simulink model "Controller_v2"  (R2015b)
settings: Solver=VariableStepAuto  StartTime=0.0  StopTime=10.0  RelTol=1e-3
settings Model: Creator=MVdB  LastModifiedBy=Niels

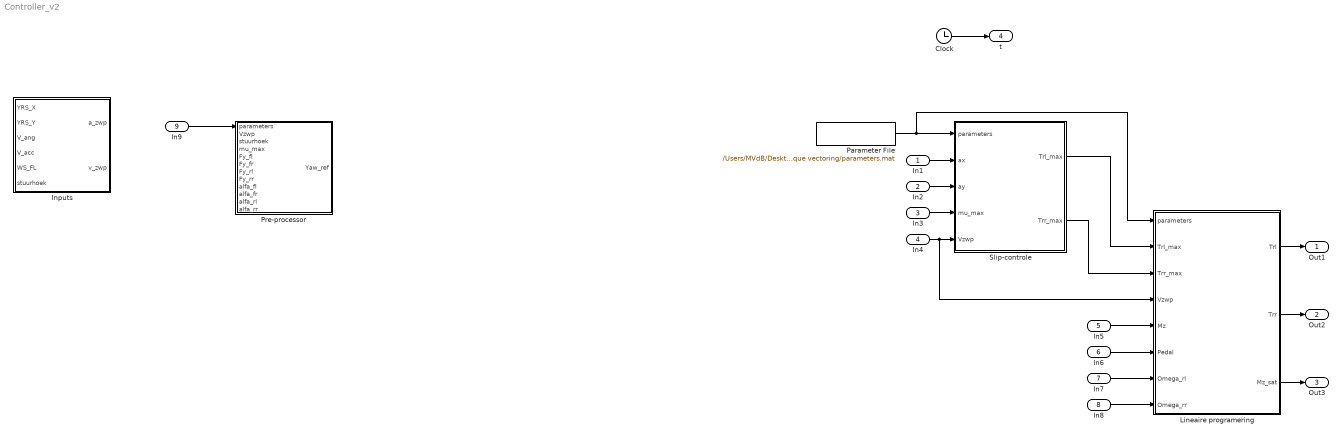
== system Controller_v2 ==
  In1 : Inport
  In2 : Inport  Port=2
  In3 : Inport  Port=3
  In4 : Inport  Port=4
  In5 : Inport  Port=5
  In6 : Inport  Port=6
  In7 : Inport  Port=7
  In8 : Inport  Port=8
  In9 : Inport  Port=9
  Clock : Clock
  Inputs : MATLAB Function  TreatAsAtomicUnit=on
  Lineaire programering : MATLAB Function  TreatAsAtomicUnit=on
  Parameter File : FromFile  FileName=/Users/MVdB/Desktop/FEB/Torque vectoring/parameters.mat  SampleTime=0
  Pre-processor : MATLAB Function  TreatAsAtomicUnit=on
  "Slip-controle " : MATLAB Function  TreatAsAtomicUnit=on
  Out1 : Outport
  Out2 : Outport  Port=2
  Out3 : Outport  Port=3
  t : Outport  Port=4
  wires:
  "Slip-controle "/2(Trr_max) -> Lineaire programering/3(Trr_max)
  "Slip-controle "/1(Trl_max) -> Lineaire programering/2(Trl_max)
  In1/1 -> "Slip-controle "/2(ax)
  In2/1 -> "Slip-controle "/3(ay)
  Lineaire programering/3(Mz_sat) -> Out3/1
  Lineaire programering/1(Trl) -> Out1/1
  Lineaire programering/2(Trr) -> Out2/1
  In3/1 -> "Slip-controle "/4(mu_max)
  In4/1 -> Lineaire programering/4(Vzwp), "Slip-controle "/5(Vzwp)
  In5/1 -> Lineaire programering/5(Mz)
  In6/1 -> Lineaire programering/6(Pedal)
  In7/1 -> Lineaire programering/7(Omega_rl)
  In8/1 -> Lineaire programering/8(Omega_rr)
  Clock/1 -> t/1
  Parameter File/1 -> Lineaire programering/1(parameters), "Slip-controle "/1(parameters)
  In9/1 -> Pre-processor/1(parameters)

== matlab function Controller_v2/Lineaire programering ==
  data: parameters input; Trl_max input; Trl output; Trr_max input; Vzwp input; Mz input; Pedal input; Omega_rl input; Omega_rr input; Trr output; Mz_sat output
function [Trl,Trr,Mz_sat] = Lineaire_programmering(parameters,Trl_max,Trr_max,Vzwp,Mz,Pedal,Omega_rl,Omega_rr)
%Deze blok staat in voor het berekenen van de te leveren torque per wiel
%aan de hand van twee lineaire doelen. Het eerste doel is het netto moment
%rond het zwaartepunt optimaliseren. Het tweede doel is de torque die wordt
%overgedragen op het wegdek optimaliseren.

%Gevraagd Moment
TV_control = (Mz*Reff_r)/(2*Sr*Gr);

TV_max_1 = min(400,((Trl_max+Trr_max)/2));


f = [Trr_1 Trl_1 e];
A = [Trr_1 Trl_1
    0];
b = [Tmax e];
Aeq = [Trr_1 -Trl_1 e];
beq = 2*max(-TV_max_1,min(TV_max_1,TV_control));
lb = [-Trr_1,-Trl_1];
ub = [Trr_1,Trl_1];

x = linprog(f,A,b,Aeq,beq,lb,ub);


%Gevraagde torque
TV_max_2 = max(0,min(400,(Trl_max-(Ttot/2)),(Trr_max+(Ttot/2))));

f_2 = [Trr_2 Trl_2];
A_2 = [Trr_2 Trl_2];
b_2 = Tmax;
Aeq_2 = [Trr_2 -Trl_2];
beq_2 = 2*max(-TV_max_2,min(TV_max_2,TV_control));
lb_2 = [-Trr_2,-Trl_2];
ub_2 = [Trr_2,Trl_2];

x_2  = linprog(f_2,A_2,b_2,Aeq_2,beq_2,lb_2,ub_2);


%Effectieve torques naar motordrives
Trl = x(2)*Cte + x_2(2)*(1-Cte);
Trr = x(1)*Cte + x_2(1)*(1-Cte);

== matlab function Controller_v2/Slip-controle  ==
  data: parameters input; ax input; ay input; mu_max input; Trl_max output; Vzwp input; Trr_max output
function [Trl_max,Trr_max] = Slip_controle(parameters,ax,ay,mu_max,Vzwp)
% Berekening van de maximale torques die men kan toepassen op de wielen
% door berekening van de normaalkrachten op de wielen.

load('parameters.mat');

%Wielbelastingen

%Statische wielbelasting
Ws_fl = (Lf/(2*L))*M*g;
Ws_fr = Ws_fl;
Ws_rl = (Lr/(2*L))*M*g;
Ws_rr = Ws_rl;

Ws_f = Ws_fl + Ws_fr;
Ws_r = Ws_rl + Ws_rr;

%Laterale wielbelasting (door rollen van de wagen)
FfsM = (Ksf*W*ay*D)/(Tf(Ksf+Ksr-(W*g*D)));   %Kracht door rolmoment
FrsM = (Ksr*W*ay*D)/(Tr(Ksf+Ksr-(W*g*D)));

FfsF = (Ws_f*ay*Hrcf)/Tf;                    %Kracht door afgeveerde massa
FrsF = (Ws_r*ay*Hrcr)/Tr;

FfuF = (Wu_f*ay*Hurcf)/Tf;                   %Kracht door onafgeveerde massa
FruF = (Wu_r*ay*Hurcr)/Tr;

Ff = FfsM + FfsF + FfuF;                    %Totale gewichtsverplaatsing
Fr = FrsM + FrsF + FruF;

Wy_fl = Ff/2;                               %Kracht per wiel
Wy_fr = -Wy_fl;
Wy_rl = Fr/2;
Wy_rr = -Wy_rl;

%Longitudinale wielbelasting
Wx_fl = (-H/(2*L))*W*ax;
Wx_fr = Wx_fl;
Wx_rl = (H/(2*L))*W*ax;
Wx_rr = Wx_rl;

%Aerodynamische wielbelasting
Wa_fl = (-LF/(2*L))+((Krf/(Krf+Krr))*(Rm/Tf));
Wa_fr = (-LF/(2*L))-((Krf/(Krf+Krr))*(Rm/Tf));
Wa_rl = (-LR/(2*L))+((Krr/(Krf+Krr))*(Rm/Tr));
Wa_rr = (-LR/(2*L))-((Krr/(Krf+Krr))*(Rm/Tr));

%anti-roll bar wielbelasting
Wab_fl = (Krf_a/((Krf_a+((Kwf*(Tf)^2)/2))*Wy_fl));
Wab_fr = -Wab_fl;
Wab_rl = (Krr_a/((Krr_a+((Kwr*(Tr)^2)/2))*Wy_rl));
Wab_rr = -Wab_rl;

%Totale belasting per wiel
Wfl = Ws_fl + Wy_fl + Wx_fl + Wa_fl + Wab_fl;   %Ongebruikt, kan later gebruikt worden voor 4WD
Wfr = Ws_fr + Wy_fr + Wx_fr + Wa_fr + Wab_fr;   %^ Idem
Wrl = Ws_rl + Wy_rl + Wx_rl + Wa_rl + Wab_rl;
Wrr = Ws_rr + Wy_rr + Wx_rr + Wa_rr + Wab_rr;



%Omrekening naar torques

%Wrijvingscirkels
Fx_rl = sqrt((Wrl^2*mu_max^2)-(Wrl^2*ay^2));
Fx_rr = sqrt((Wrr^2*mu_max^2)-(Wrr^2*ay^2));

%Maximum torques
Trl_max = Fx_rl*Reff_r;
Trr_max = Fx_rr*Reff_r;

== matlab function Controller_v2/Pre-processor ==
  data: parameters input; Yaw_ref output; Vzwp input; stuurhoek input; mu_max input; Fy_fl input; Fy_fr input; Fy_rl input; Fy_rr input; alfa_fl input; alfa_fr input; alfa_rl input; alfa_rr input
function Yaw_ref = pre_processor(parameters,Vzwp,stuurhoek,mu_max,Fy_fl,Fy_fr,Fy_rl,Fy_rr,alfa_fl,alfa_fr,alfa_rl,alfa_rr)
%De pre-processor berekend de gewenste yaw rate door het minimum te nemen
%van de ideale en de maximale yaw rate waarde.

%Berekening massa's
Mf = M*(Lr/L);
Mr = M*(Lf/L);

%Berekening Cornering stiffness
C_fl = (Fy_fl/alfa_fl);
C_fr = (Fy_fr/alfa_fr);
C_rl = (Fy_rl/alfa_rl);
C_rr = (Fy_rr/alfa_rr);

%Gemiddelde van de cornering stiffness vooraan en achteraan nemen
 Cf = ((C_fl + C_fr)/ 2);
 Cr = ((C_rl + C_rr)/ 2);
%Berekening van de onderstuur factor.
Ku = ((Mf/Cf)-(Mr/Cr));

%Berekening van de ideale yaw rate.
Yaw_id = ((Vzwp*stuurhoek)/((Lf+Lr)+Ku*(Vzwp)^2));

% berekening van de sliphoek beita
beita = atan(Lf * tan(stuurhoek)/ (Lf+Lr)) ;

%Berekening van de maximale yaw rate.
Yaw_max = ((mu_max*g)/(Vzwp*cos(beita)))-Vzwp*diff(beita)*cos(beita);

%Minimale yaw rate.
Yaw_ref = min(Yaw_id,Yaw_max);

== matlab function Controller_v2/Inputs ==
  data: YRS_X input; YRS_Y input; V_ang input; V_acc input; WS_FL input; a_zwp output; v_zwp output; stuurhoek input
function [a_zwp,v_zwp]= Inputs(YRS_X,YRS_Y,V_ang,V_acc,WS_FL,stuurhoek)
% hier zullen de inputs verwrkt worden die nodig zijn voor de aansturing van het controle algortihme
    % YRS is de versnelling die gemeten word door de yaw-rate sensor
    % V_ang is de hoeksnelheid       
    % V_acc is de hoekversnelling
% berekening van de versnelling van het zwaartepunt in de x-richting
a_zwpx = YRS_X + (V_acc *R2) + V_ang*(V_ang*R1);

% versnelling in de y-richting
a_zwpy = YRS_Y + (V_acc *R1) + V_ang*(V_ang*R2);

% Totale versnelling van het zwaartepunt
a_zwp = square ((a_zwpx^2) + (a_zwpy^2)); 
    
% De snelheid van het zwaartepunt
C = 0;                                           % beginconditie integratieterm = 0 
while do 

   v_zwpacc = integrate ( a_zwp)+ C;              % C is de beginsnelheid
    C = v_zwpacc;
end   
    % De snelheid op bassis van de wielspeed sensoren 
    % V_FL is de snelheid van het linker voorwiel, WS_FL is de hoeksnelheid van
    % dit wiel en R3 is de banden straal
    
V_FL = WS_FL * Reff;
v_zwpwiel = V_FL *cos(stuurhoek)+ V_FL * sin (stuurhoek) + V_ang * (R4_x - R4_y);

 % vergelijken van deze twee snelheden
 
 if (v_zwpwiel- v_zwpacc)> -0.05   && (v_zwpwiel- v_zwpacc)< 0.05 
     then      v_zwp = v_zwpwiel                                 % wagen slipt niet
 else
                                                           % wagen slipt                                                                % slipt
                                                               
 end
